simulink model "rlsuspension"  (R2023a)
settings: Solver=VariableStepAuto  StartTime=0.0  StopTime=5  RelTol=1e-3
libraries: simulink x6, rllib x1
settings Model: Creator=Abdulrahman Hamdy  LastModifiedBy=Abdulrahman Hamdy

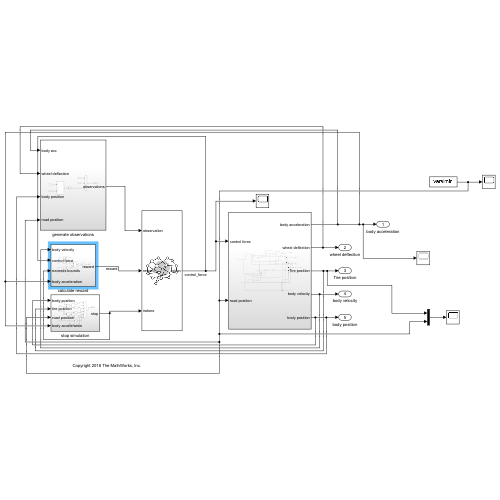
[thumbnail: Simulink's stored preview of the top-level diagram]
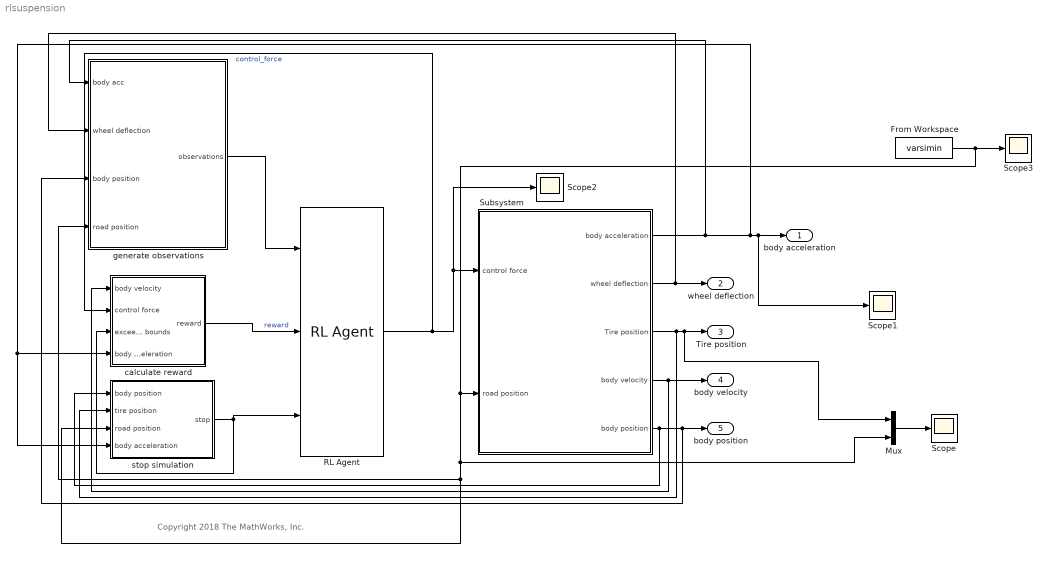
== system rlsuspension ==
  note: Copyright 2018 The MathWorks, Inc.
  From Workspace : FromWorkspace  VariableName=varsimin  SampleTime=0.01
  Mux : Mux  Inputs=2
  RL Agent : rllib/RL Agent  Agent=agent  ExternalActionAsInput=off  ProvideLastAction=off  ProvideCumRwd=off  TreatAsDirectFeedthrough=on  UseStrictObservationDataTypes=off
  Scope{,1..3} (4 alike) : Scope
  Subsystem : Subsystem
  calculate reward : Subsystem
  generate observations : Subsystem
  stop simulation : Subsystem
  body acceleration : Outport
  wheel deflection : Outport  Port=2
  Tire position : Outport  Port=3
  body velocity : Outport  Port=4
  body position : Outport  Port=5
  wires:
  stop simulation/1(stop) -> calculate reward/3(exceeds bounds), RL Agent/3
  calculate reward/1(reward) -> RL Agent/2  "reward"
  generate observations/1(observations) -> RL Agent/1
  RL Agent/1 -> calculate reward/2(control force), Subsystem/1(control force), Scope2/1  "control_force"
  Subsystem/1(body acceleration) -> generate observations/1(body acc), Scope1/1, body acceleration/1, calculate reward/4(body acceleration), stop simulation/4(body acceleration)
  Subsystem/2(wheel deflection) -> generate observations/2(wheel deflection), wheel deflection/1
  Subsystem/3(Tire position) -> stop simulation/2(tire position), Mux/1, Tire position/1
  Subsystem/4(body velocity) -> calculate reward/1(body velocity), body velocity/1
  Subsystem/5(body position) -> stop simulation/1(body position), generate observations/3(body position), body position/1
  From Workspace/1 -> Mux/2, stop simulation/3(road position), generate observations/4(road position), Subsystem/2(road position), Scope3/1
  Mux/1 -> Scope/1

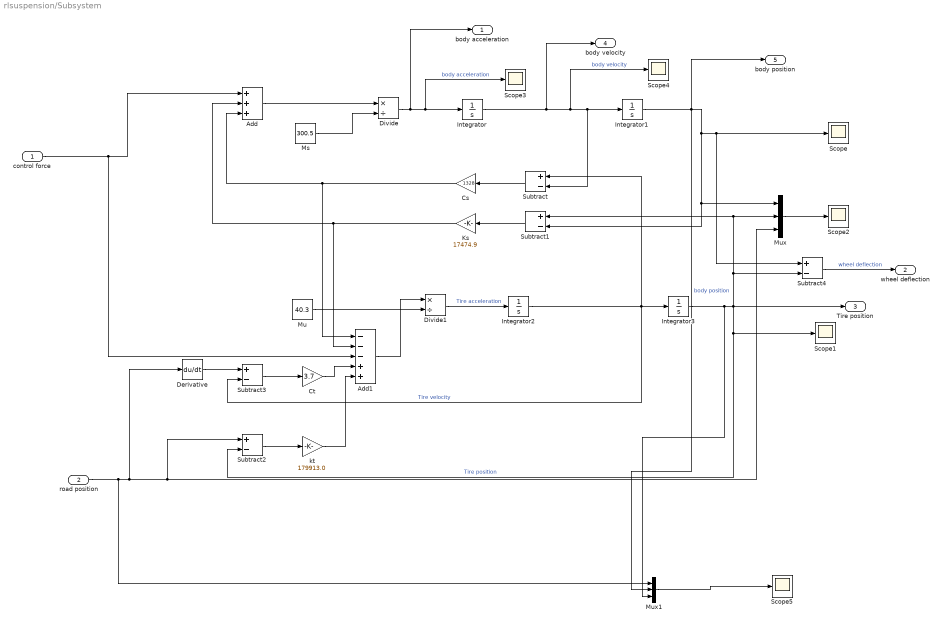
== system rlsuspension/Subsystem ==
  control force : Inport
  road position : Inport  Port=2
  Add : Sum  Inputs=+++
  Add1 : Sum  Inputs=---++
  Cs : Gain  Gain=1328
  Ct : Gain  Gain=3.7
  Derivative : Derivative
  Divide : Product  Inputs=*/
  Divide1 : Product  Inputs=*/
  Integrator{,1..3} (4 alike) : Integrator
  Ks : Gain  Gain=17474.9
  Ms : Constant  Value=300.5
  Mu : Constant  Value=40.3
  Mux : Mux  Inputs=3
  Mux1 : Mux  Inputs=3
  Scope{,1..5} (6 alike) : Scope
  Subtract{,1..4} (5 alike) : Sum  Inputs=+-
  kt : Gain  Gain=179913.0
  body acceleration : Outport
  wheel deflection : Outport  Port=2
  Tire position : Outport  Port=3
  body velocity : Outport  Port=4
  body position : Outport  Port=5
  wires:
  Ms/1 -> Divide/2
  Integrator1/1 -> body position/1, Mux1/2, Mux/1, Subtract1/2, Scope/1, Subtract4/1  "body position"
  Integrator2/1 -> Subtract/1, Subtract3/2, Integrator3/1  "Tire velocity"
  Integrator3/1 -> Mux1/3, Tire position/1, Subtract4/2, Mux/2, Subtract1/1, Scope1/1, Subtract2/2  "Tire position"
  Ks/1 -> Add1/2, Add/2
  Ct/1 -> Add1/4
  Integrator/1 -> body velocity/1, Scope4/1, Subtract/2, Integrator1/1  "body velocity"
  road position/1 -> Mux1/1, Derivative/1, Subtract2/1, Mux/3
  Subtract3/1 -> Ct/1
  control force/1 -> Add1/3, Add/1
  Divide/1 -> body acceleration/1, Scope3/1, Integrator/1  "body acceleration"
  Cs/1 -> Add1/1, Add/3
  Add1/1 -> Divide1/1
  Add/1 -> Divide/1
  kt/1 -> Add1/5
  Mu/1 -> Divide1/2
  Divide1/1 -> Integrator2/1  "Tire acceleration"
  Derivative/1 -> Subtract3/1
  Mux1/1 -> Scope5/1
  Subtract1/1 -> Ks/1
  Subtract/1 -> Cs/1
  Mux/1 -> Scope2/1
  Subtract2/1 -> kt/1
  Subtract4/1 -> wheel deflection/1  "wheel deflection"

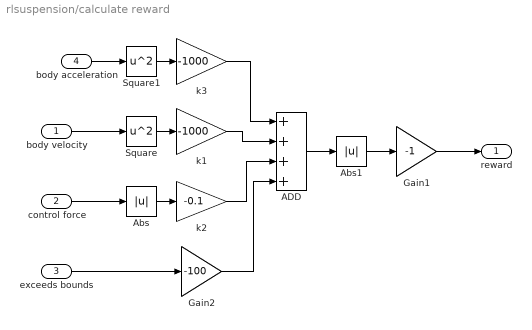
== system rlsuspension/calculate reward ==
  body velocity : Inport
  control force : Inport  Port=2
  exceeds bounds : Inport  Port=3
  body acceleration : Inport  Port=4
  ADD : Sum  Inputs=++++
  Abs : Abs  SaturateOnIntegerOverflow=off
  Abs1 : Abs  SaturateOnIntegerOverflow=off
  Gain1 : Gain  Gain=-1
  Gain2 : Gain  Gain=-100
  Square : Math  Operator=square
  Square1 : Math  Operator=square
  k1 : Gain  Gain=-1000
  k2 : Gain  Gain=-0.1
  k3 : Gain  Gain=-1000
  reward : Outport  VectorParamsAs1DForOutWhenUnconnected=off
  wires:
  Abs/1 -> k2/1
  exceeds bounds/1 -> Gain2/1
  control force/1 -> Abs/1
  body velocity/1 -> Square/1
  Square/1 -> k1/1
  body acceleration/1 -> Square1/1
  Square1/1 -> k3/1
  k3/1 -> ADD/1
  k1/1 -> ADD/2
  k2/1 -> ADD/3
  Gain2/1 -> ADD/4
  ADD/1 -> Abs1/1
  Gain1/1 -> reward/1
  Abs1/1 -> Gain1/1

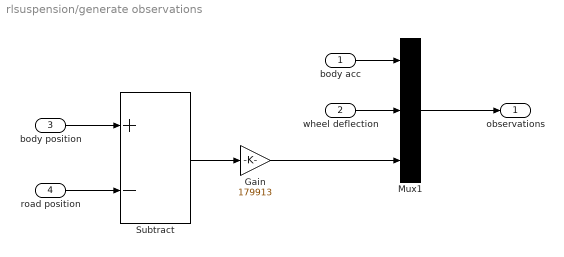
== system rlsuspension/generate observations ==
  body acc : Inport
  wheel deflection : Inport  Port=2
  body position : Inport  Port=3
  road position : Inport  Port=4
  Gain : Gain  Gain=179913
  Mux1 : Mux  Inputs=3
  Subtract : Sum  Inputs=+-
  observations : Outport  VectorParamsAs1DForOutWhenUnconnected=off
  wires:
  body acc/1 -> Mux1/1
  wheel deflection/1 -> Mux1/2
  body position/1 -> Subtract/1
  road position/1 -> Subtract/2
  Subtract/1 -> Gain/1
  Gain/1 -> Mux1/3
  Mux1/1 -> observations/1

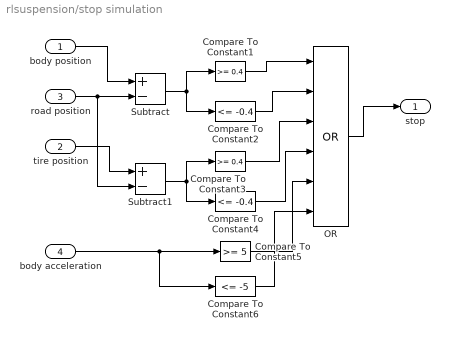
== system rlsuspension/stop simulation ==
  body position : Inport
  tire position : Inport  Port=2
  road position : Inport  Port=3
  body acceleration : Inport  Port=4
  Compare To Constant1 : simulink/Logic and Bit Operations/Compare To Constant  relop=>=  const=0.4  OutDataTypeStr=boolean
  Compare To Constant2 : simulink/Logic and Bit Operations/Compare To Constant  relop=<=  const=-0.4  OutDataTypeStr=boolean
  Compare To Constant3 : simulink/Logic and Bit Operations/Compare To Constant  relop=>=  const=0.4  OutDataTypeStr=boolean
  Compare To Constant4 : simulink/Logic and Bit Operations/Compare To Constant  relop=<=  const=-0.4  OutDataTypeStr=boolean
  Compare To Constant5 : simulink/Logic and Bit Operations/Compare To Constant  relop=>=  const=5  OutDataTypeStr=boolean
  Compare To Constant6 : simulink/Logic and Bit Operations/Compare To Constant  relop=<=  const=-5  OutDataTypeStr=boolean
  OR : Logic  Operator=OR  Inputs=6  IconShape=distinctive  AllPortsSameDT=off  OutDataTypeStr=boolean
  Subtract : Sum  Inputs=+-
  Subtract1 : Sum  Inputs=+-
  stop : Outport  VectorParamsAs1DForOutWhenUnconnected=off
  wires:
  Compare To Constant2/1 -> OR/2
  Compare To Constant1/1 -> OR/1
  OR/1 -> stop/1
  body position/1 -> Subtract/1
  Subtract/1 -> Compare To Constant1/1, Compare To Constant2/1
  tire position/1 -> Subtract1/1
  road position/1 -> Subtract1/2, Subtract/2
  Subtract1/1 -> Compare To Constant3/1, Compare To Constant4/1
  Compare To Constant3/1 -> OR/3
  Compare To Constant4/1 -> OR/4
  body acceleration/1 -> Compare To Constant6/1, Compare To Constant5/1
  Compare To Constant5/1 -> OR/5
  Compare To Constant6/1 -> OR/6
